simulink model "Diode_Clamped_Multilevel_Inverter"  (R2024a)
settings: Solver=FixedStepAuto  StartTime=0.0  StopTime=2/fe  FixedStep=1/(100*fsw)  RelTol=1e-3
values from neighbouring files (symbols this model uses):
  B = 0*0.0025    (= 0)    [ECE_598_script_file.m]
  fe = 100    [ECE_598_script_file.m]
  fsw = 1000    [ECE_598_script_file.m]
  J = 0.01    [ECE_598_script_file.m]
  Lrl_dash = 9.6e-3    (= 0.0096)    [ECE_598_script_file.m]
  Lsl = 9.6e-3    (= 0.0096)    [ECE_598_script_file.m]
  M = 165e-3    (= 0.165)    [ECE_598_script_file.m]
  Rr = 4.23    [ECE_598_script_file.m]
  Rs = 3.57    [ECE_598_script_file.m]
  tau_L = 2    [ECE_598_script_file.m]
  turns_ratio = 0.682    [ECE_598_script_file.m]
  Vdc = 400    [ECE_598_script_file.m]
  Vm = 200    [ECE_598_script_file.m]
undefined symbols (not defined in the file or in its folder): j, jsin
libraries: nesl_utility x23, ee_lib x20, fl_lib x12
(part 1 of 2)
settings Model: Creator=dm69  LastModifiedBy=dm69

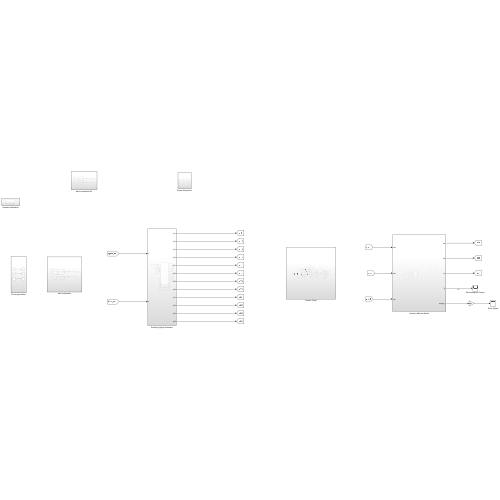
[thumbnail: Simulink's stored preview of the top-level diagram]
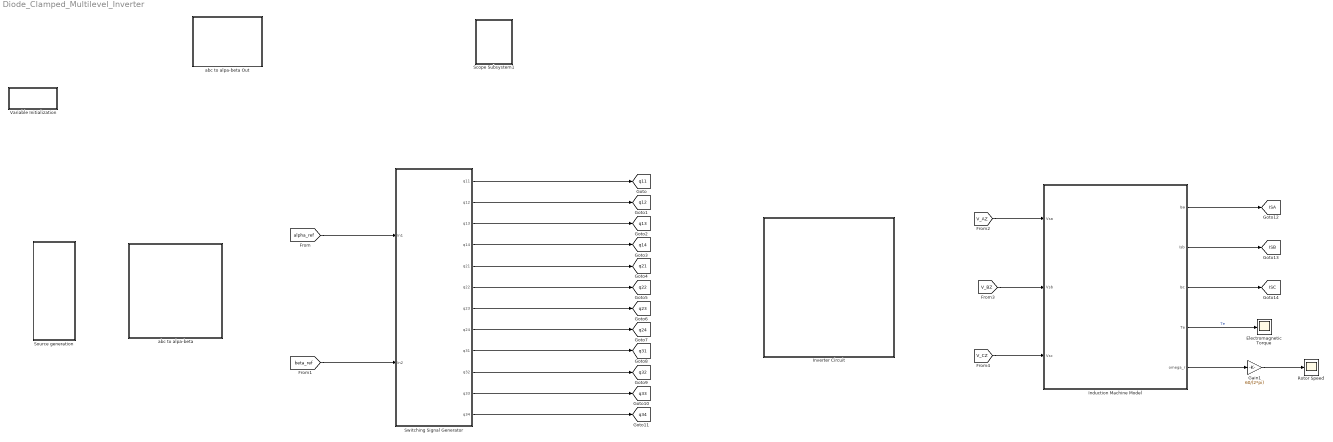
== system Diode_Clamped_Multilevel_Inverter ==
  Electromagnetic Torque : Scope
  Gain1 : Gain  Gain=60/(2*pi)
  Induction Machine Model : Subsystem
  Inverter Circuit : Subsystem
  Rotor Speed : Scope
  Scope Subsystem1 : Subsystem
  Source generation : Subsystem
  Switching Signal Generator : Subsystem
  Variable Initialization : Subsystem
  abc to alpa-beta : Subsystem
  abc to alpa-beta Out : Subsystem
  tag scope: ISA=global, ISB=global, ISC=global, q11=global, q12=global, q13=global, q14=global, q21=global, q22=global, q23=global, q24=global, q31=global, q32=global, q33=global, q34=global
  wires:
  Gain1/1 -> Rotor Speed/1
  Induction Machine Model/2(Isb) -> [ISB]
  Induction Machine Model/3(Isc) -> [ISC]
  Induction Machine Model/1(Isa) -> [ISA]
  Switching Signal Generator/11(q33) -> [q33]
  Switching Signal Generator/12(q34) -> [q34]
  Switching Signal Generator/10(q32) -> [q32]
  Switching Signal Generator/8(q24) -> [q24]
  Switching Signal Generator/9(q31) -> [q31]
  Switching Signal Generator/6(q22) -> [q22]
  Induction Machine Model/5(omega_r) -> Gain1/1
  Switching Signal Generator/3(q13) -> [q13]
  Switching Signal Generator/2(q12) -> [q12]
  Switching Signal Generator/1(q11) -> [q11]
  Switching Signal Generator/4(q14) -> [q14]
  Switching Signal Generator/5(q21) -> [q21]
  [alpha_ref] -> Switching Signal Generator/1(In1)
  Induction Machine Model/4(Te) -> Electromagnetic Torque/1  "Te"
  [beta_ref] -> Switching Signal Generator/2(In2)
  Switching Signal Generator/7(q23) -> [q23]
  [V_AZ] -> Induction Machine Model/1(Vsa)
  [V_BZ] -> Induction Machine Model/2(Vsb)
  [V_CZ] -> Induction Machine Model/3(Vsc)

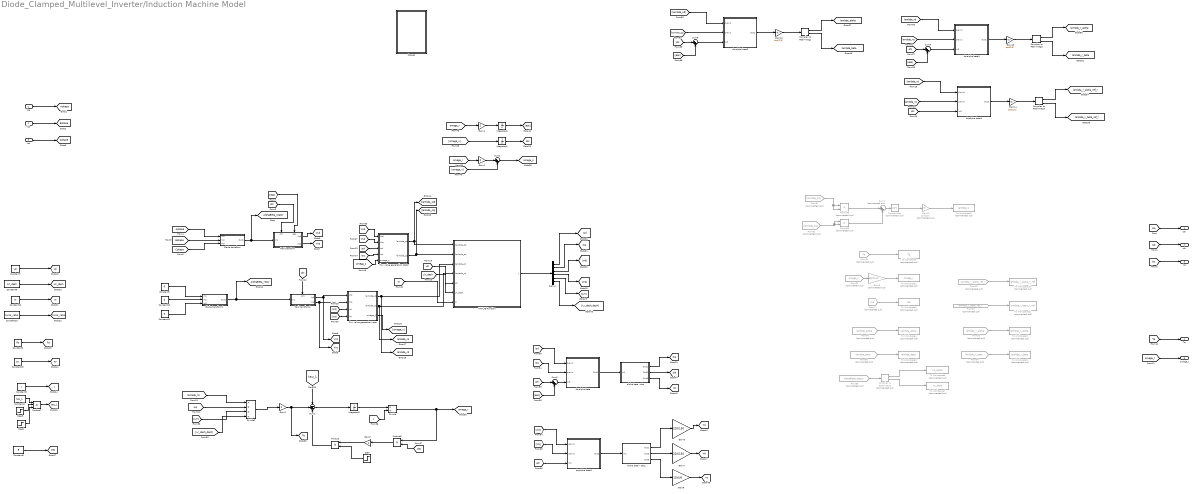
== system Diode_Clamped_Multilevel_Inverter/Induction Machine Model ==
  Vsa : Inport
  Vsb : Inport  Port=2
  Vsc : Inport  Port=3
  Clarke transform : Subsystem
  Clarke transform1 : Subsystem
  Complex to Real-Imag1 : ComplexToRealImag
  Complex to Real-Imag2 : ComplexToRealImag  Commented=on
  Complex to Real-Imag3 : ComplexToRealImag
  Complex to Real-Imag4 : ComplexToRealImag
  Constant10 : Constant  Value=0
  Constant11 : Constant  Value=0
  Constant12 : Constant  Value=M
  Constant13 : Constant  Value=turns_ratio
  Constant15 : Constant  Value=Rr
  Constant3 : Constant  Value=J
  Constant4 : Constant  Value=tau_L
  Constant5 : Constant  Value=Rs
  Constant6 : Constant  Value=B
  Constant7 : Constant  Value=Lsl
  Constant8 : Constant  Value=Lrl_dash
  Constant9 : Constant  Value=0
  Demux : Demux  Outputs=6
  Divide : Product  Inputs=*/
  Divide2 : Product  Inputs=***/
  From43 : From  Commented=on  GotoTag=lambda_r_alpha_ref_r  TagVisibility=global
  From61 : From  Commented=on  GotoTag=Te  TagVisibility=global
  From62 : From  Commented=on  GotoTag=omega_r
  From74 : From  Commented=on  GotoTag=Isa  TagVisibility=global
  From81 : From  Commented=on  GotoTag=lambda_sd
  From82 : From  Commented=on  GotoTag=lambda_sq
  From87 : From  Commented=on  GotoTag=lambda_alpha  TagVisibility=global
  From88 : From  Commented=on  GotoTag=lambda_beta  TagVisibility=global
  From89 : From  Commented=on  GotoTag=AlphaBeta_stator
  From92 : From  Commented=on  GotoTag=lambda_r_beta_ref_r  TagVisibility=global
  From93 : From  Commented=on  GotoTag=lambda_r_alpha  TagVisibility=global
  From94 : From  Commented=on  GotoTag=lambda_r_beta  TagVisibility=global
  Gain1 : Gain  Gain=2
  Gain11 : Gain  Commented=on  Gain=sqrt(2/3)
  Gain12 : Gain  Gain=sqrt(2/3)
  Gain13 : Gain  Gain=sqrt(2/3)
  Gain14 : Gain  Gain=sqrt(2/3)
  Gain2 : Gain  Gain=2
  Gain3 : Gain
  Gain4 : Gain  Gain=2
  Gain6 : Gain  Gain=220/150
  Gain7 : Gain  Gain=220/150
  Gain8 : Gain  Gain=220/150
  Gain9 : Gain  Commented=on  Gain=60/(2*pi)
  Integrator1 : Integrator  InitialCondition=1e-4
  Integrator3 : Integrator
  Integrator6 : Integrator  InitialCondition=1e-4
  MATLAB Function : MATLAB Function  TreatAsAtomicUnit=on
  Park transform : Subsystem
      settings: PortSchema="{\"entries\":[{\"content\":{\"sides\":[{\"content\":{\"connectorIds\":[\"In1\"]},\"type\":\"ConnectorPlacement.EquallySpacedRectSide\",\"uuid\":\"6c71d13c-178f-4a42-b33e-304e9d2b6e08\"},{\"content\":{\"connectorIds\":[\"Out1\",\"Out2\"],\"side\":\"RIGHT\"},\"type\":\"ConnectorPlacement.EquallySpacedRectSide\",\"uuid\":\"2a6462c8-5182-4726-b418-a85255dbc142\"},{\"content\":{\"connectorIds\":[\"In2\",\"In3\"],\"side\":\"TOP\"},\"type\":\"ConnectorPlacement.EquallySpacedRectSide\",\"uuid\":\"09083f92-b28e-408e-9b2d-669b336a5b1a\"}]},\"type\":\"ConnectorPlacement.EquallySpacedConnector\",\"uuid\":\"431009d8-f15a-4fdd-ac9b-0312528d9d69\"}],\"packageUris\":[\"http://schema.mathworks.com/mf0/Connector/R2020b\"],\"version\":\"1.0\"}"
  Park transform1 : Subsystem
      settings: PortSchema="{\"entries\":[{\"content\":{\"sides\":[{\"content\":{\"connectorIds\":[\"In1\"]},\"type\":\"ConnectorPlacement.EquallySpacedRectSide\",\"uuid\":\"6c71d13c-178f-4a42-b33e-304e9d2b6e08\"},{\"content\":{\"connectorIds\":[\"Out1\",\"Out2\"],\"side\":\"RIGHT\"},\"type\":\"ConnectorPlacement.EquallySpacedRectSide\",\"uuid\":\"2a6462c8-5182-4726-b418-a85255dbc142\"},{\"content\":{\"connectorIds\":[\"In2\"],\"side\":\"TOP\"},\"type\":\"ConnectorPlacement.EquallySpacedRectSide\",\"uuid\":\"09083f92-b28e-408e-9b2d-669b336a5b1a\"}]},\"type\":\"ConnectorPlacement.EquallySpacedConnector\",\"uuid\":\"431009d8-f15a-4fdd-ac9b-0312528d9d69\"}],\"packageUris\":[\"http://schema.mathworks.com/mf0/Connector/R2020b\"],\"version\":\"1.0\"}"
  Product : Product
  Product2 : Product
  Product7 : Product  Inputs=3
  Product8 : Product  Commented=on
  Product9 : Product  Commented=on
  Scopes : Subsystem
  Square Root : Sqrt  Commented=on
  Step : Step  Time=1e-3  SampleTime=0
  Step1 : Step  Time=8  Before=1  After=0  SampleTime=0
  Step3 : Step  Time=4  SampleTime=0
  Sum1 : Sum  Inputs=-+-
  Sum{2,5,8..9} (4 alike) : Sum  Inputs=|++
  Sum7 : Sum  Commented=on  Inputs=|++
  To Workspace : ToWorkspace  Commented=on  VariableName=Te  SaveFormat=Timeseries  SampleTime=-1
  To Workspace1 : ToWorkspace  Commented=on  VariableName=omega_r  SaveFormat=Timeseries  SampleTime=-1
  To Workspace10 : ToWorkspace  Commented=on  VariableName=lambda_r_alpha_r_ref  SaveFormat=Timeseries  SampleTime=-1
  To Workspace11 : ToWorkspace  Commented=on  VariableName=lambda_r_beta_r_ref  SaveFormat=Timeseries  SampleTime=-1
  To Workspace2 : ToWorkspace  Commented=on  VariableName=Isa  SaveFormat=Timeseries  SampleTime=-1
  To Workspace3 : ToWorkspace  Commented=on  VariableName=lambda_s  SaveFormat=Timeseries  SampleTime=-1
  To Workspace4 : ToWorkspace  Commented=on  VariableName=lambda_alpha  SaveFormat=Timeseries  SampleTime=-1
  To Workspace5 : ToWorkspace  Commented=on  VariableName=lambda_beta  SaveFormat=Timeseries  SampleTime=-1
  To Workspace6 : ToWorkspace  Commented=on  VariableName=Vs_alpha  SaveFormat=Timeseries  SampleTime=-1
  To Workspace7 : ToWorkspace  Commented=on  VariableName=Vs_beta  SaveFormat=Timeseries  SampleTime=-1
  To Workspace8 : ToWorkspace  Commented=on  VariableName=lambda_r_alpha  SaveFormat=Timeseries  SampleTime=-1
  To Workspace9 : ToWorkspace  Commented=on  VariableName=lambda_r_beta  SaveFormat=Timeseries  SampleTime=-1
  alpha beta - abc : Subsystem
  alpha beta - abc1 : Subsystem
  dq-alpha beta : Subsystem
  dq-alpha beta1 : Subsystem
  dq-alpha beta2 : Subsystem
  dq-alpha beta3 : Subsystem
  dq-alpha beta4 : Subsystem
  flux value generation rotor : Subsystem
  flux value generation stator : Subsystem
  Isa : Outport
  Isb : Outport  Port=2
  Isc : Outport  Port=3
  Te : Outport  Port=4
  omega_r : Outport  Port=5
  tag scope: AlphaBeta_rotor=global, AlphaBeta_stator=global, Aphase=global, Bphase=global, Cphase=global, Ira=global, Irb=global, Irc=global, Isa=global, Isb=global, Isc=global, Isd=global, Isq=global, J=global, Llr_dash=global, Lsl=global, M=global, Rr=global, Rs=global, Te=global, Vrd=global, Vrq=global, Vsd=global, Vsq=global, lambda_alpha=global, lambda_beta=global, lambda_r_alpha=global, lambda_r_alpha_ref_r=global, lambda_r_beta=global, lambda_r_beta_ref_r=global, lambda_rd=global, lambda_rq=global, omega_r=global, omega_s=global, phi=global, tau_L=global, turns_ratio=global
  wires:
  Gain4/1 -> Integrator6/1
  Clarke transform/1(Out1) -> [AlphaBeta_stator], Park transform/1(In1)
  Constant9/1 -> Clarke transform1/1(In1)
  From94/1 -> To Workspace9/1
  Demux/3 -> [Ird]
  Constant8/1 -> [Llr_dash]
  Constant11/1 -> Clarke transform1/3(In3)
  Integrator1/1 -> [phi]
  Clarke transform1/1(Out1) -> [AlphaBeta_rotor], Park transform1/1(In1)
  From61/1 -> To Workspace/1
  [phi] -> Sum9/1
  Demux/5 -> [Lm]
  Gain13/1 -> Complex to Real-Imag3/1
  Gain1/1 -> Sum2/1
  [Bphase] -> Clarke transform/2(In2)
  Gain9/1 -> To Workspace1/1
  flux value generation rotor/3(omega_X) -> [omega_x]
  [Isq] -> Divide2/2
  [M] -> MATLAB Function/7(M)
  Constant10/1 -> Clarke transform1/2(In2)
  flux value generation rotor/2(lambda_rq) -> MATLAB Function/4(lambda_rq), [lambda_rq]
  [lambda_rd] -> dq-alpha beta3/1(d-axis)
  dq-alpha beta/1(Out1) -> alpha beta - abc/1(In1)
  [Lr_dash_dash] -> Divide2/4
  [phi] -> dq-alpha beta1/3(In1)
  Constant15/1 -> [Rr]
  [Aphase] -> Clarke transform/1(In1)
  Complex to Real-Imag3/2 -> [lambda_r_beta]
  Integrator6/1 -> [eps]
  [Cphase] -> Clarke transform/3(In3)
  [Llr_dash] -> MATLAB Function/6(Lrl_dash)
  Sum9/1 -> dq-alpha beta3/3(In3)
  [omega_r] -> Gain1/1
  Gain6/1 -> [Ira]
  Park transform1/2(Vrq) -> [Vrq], flux value generation rotor/2(Vrq)
  Gain2/1 -> [Te], Sum1/2
  dq-alpha beta1/1(Out1) -> alpha beta - abc1/1(In1)
  alpha beta - abc1/1(Out1) -> Gain6/1
  [omega_s] -> flux value generation stator/5(omega_s)
  Constant5/1 -> [Rs]
  [lambda_rq] -> dq-alpha beta3/2(q-axis)
  flux value generation rotor/1(lambda_rd) -> MATLAB Function/3(lambda_rd), [lambda_rd]
  [eps] -> Park transform/3(eps)
  From81/1 -> Product8/2, Product8/1
  [J] -> Divide/2
  Sum1/1 -> Integrator3/1
  From88/1 -> To Workspace5/1
  Product7/1 -> [tau_L]
  [Lsl] -> MATLAB Function/5(Lsl)
  Demux/1 -> [Isd]
  Complex to Real-Imag4/2 -> [lambda_r_beta_ref_r]
  MATLAB Function/1(y) -> Demux/1
  alpha beta - abc/2(Out2) -> [Isb]
  [lambda_rd] -> Divide2/1
  Gain11/1 -> To Workspace3/1
  [B] -> Product2/2
  From93/1 -> To Workspace8/1
  Demux/2 -> [Isq]
  [Isd] -> flux value generation stator/3(Isd)
  [omega_r] -> Gain4/1
  flux value generation stator/1(lambda_sd) -> [lambda_sd], MATLAB Function/1(lambda_sd)
  [lambda_sd] -> dq-alpha beta2/1(d-axis)
  [Lm] -> Divide2/3
  Park transform1/1(Vrd) -> flux value generation rotor/1(Vrd), [Vrd]
  Constant13/1 -> [turns_ratio]
  [Ird] -> flux value generation rotor/3(Ird)
  Product8/1 -> Sum7/1
  From87/1 -> To Workspace4/1
  Product2/1 -> Gain3/1
  [Vsq] -> flux value generation stator/2(Vsq)
  Divide2/1 -> Gain2/1
  [phi] -> Sum5/1
  Constant3/1 -> [J]
  [eps] -> Sum5/2
  Gain7/1 -> [Irb]
  Constant7/1 -> [Lsl]
  Product9/1 -> Sum7/2
  Sum2/1 -> [omega_s]
  [tau_L] -> Sum1/1
  flux value generation stator/2(lambda_sq) -> [lambda_sq], MATLAB Function/2(lambda_sq)
  [phi] -> Park transform1/2(phi)
  [Irq] -> dq-alpha beta1/2(q-axis)
  Gain8/1 -> [Irc]
  [omega_x] -> Integrator1/1
  [Ird] -> dq-alpha beta1/1(d-axis)
  Constant12/1 -> [M]
  alpha beta - abc/1(Out1) -> [Isa]
  Square Root/1 -> Gain11/1
  alpha beta - abc1/3(Out3) -> Gain8/1
  [eps] -> Sum9/2
  Sum5/1 -> dq-alpha beta/3(In3)
  Park transform/2(Vsq) -> [Vsq]
  From74/1 -> To Workspace2/1
  [phi] -> Sum8/1
  Sum8/1 -> dq-alpha beta2/3(In3)
  Park transform/1(Vsd) -> [Vsd]
  Sum7/1 -> Square Root/1
  [Vsd] -> flux value generation stator/1(Vsd)
  From62/1 -> Gain9/1
  From89/1 -> Complex to Real-Imag2/1
  [omega_x] -> Sum2/2
  [eps] -> Sum8/2
  dq-alpha beta2/1(Out1) -> Gain12/1
  Complex to Real-Imag1/2 -> [lambda_beta]
  [Isd] -> dq-alpha beta/1(d-axis)
  Complex to Real-Imag2/1 -> To Workspace6/1
  Step3/1 -> Product7/2
  alpha beta - abc/3(Out3) -> [Isc]
  From82/1 -> Product9/1, Product9/2
  Complex to Real-Imag1/1 -> [lambda_alpha]
  [phi] -> Park transform/2(phi)
  Demux/4 -> [Irq]
  dq-alpha beta3/1(Out1) -> Gain13/1
  Gain12/1 -> Complex to Real-Imag1/1
  dq-alpha beta4/1(Out1) -> Gain14/1
  Divide/1 -> [omega_r], Product2/1
  [Isq] -> flux value generation stator/4(Isq)
  alpha beta - abc1/2(Out2) -> Gain7/1
  Gain14/1 -> Complex to Real-Imag4/1
  [lambda_rq] -> dq-alpha beta4/2(q-axis)
  [lambda_rd] -> dq-alpha beta4/1(d-axis)
  Integrator3/1 -> Divide/1
  Complex to Real-Imag3/1 -> [lambda_r_alpha]
  Demux/6 -> [Lr_dash_dash]
  [Irq] -> flux value generation rotor/4(Irq)
  Constant6/1 -> [B]
  Constant4/1 -> Product7/1
  Complex to Real-Imag2/2 -> To Workspace7/1
  [Isq] -> dq-alpha beta/2(q-axis)
  [lambda_sq] -> dq-alpha beta2/2(q-axis)
  From92/1 -> To Workspace11/1
  [phi] -> dq-alpha beta4/3(In3)
  Complex to Real-Imag4/1 -> [lambda_r_alpha_ref_r]
  From43/1 -> To Workspace10/1
  [Isa] -> Isa/1
  [Isb] -> Isb/1
  [Isc] -> Isc/1
  [Te] -> Te/1
  [omega_r] -> omega_r/1
  Vsa/1 -> [Aphase]
  Vsb/1 -> [Bphase]
  Vsc/1 -> [Cphase]
  Gain3/1 -> Product/1
  Product/1 -> Sum1/3
  Step/1 -> Product/2
  Step1/1 -> Product7/3

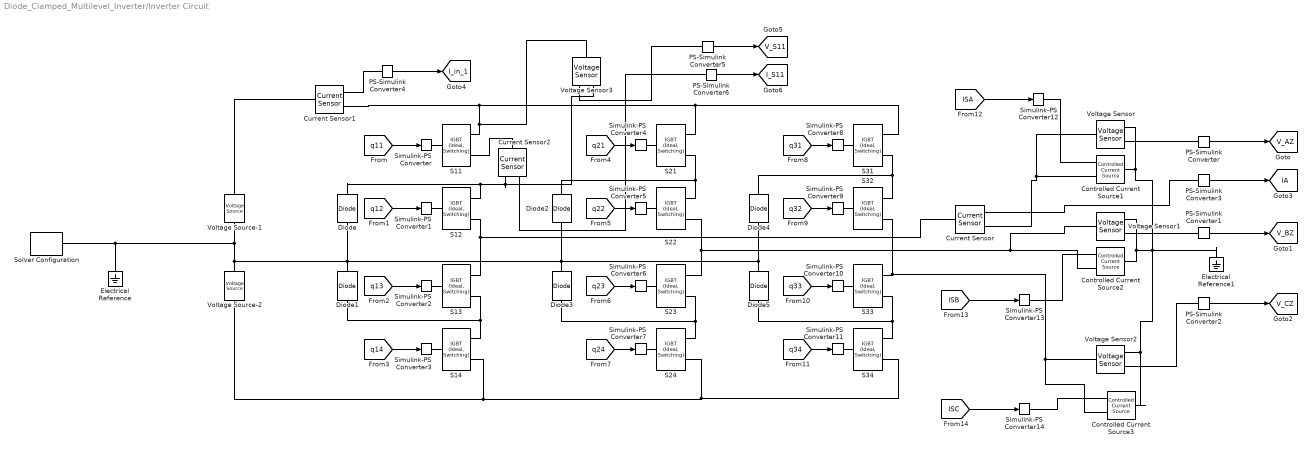
== system Diode_Clamped_Multilevel_Inverter/Inverter Circuit ==
  Controlled Current Source1 : fl_lib/Electrical/Electrical Sources/Controlled Current Source
  Controlled Current Source2 : fl_lib/Electrical/Electrical Sources/Controlled Current Source
  Controlled Current Source3 : fl_lib/Electrical/Electrical Sources/Controlled Current Source
  Current Sensor : fl_lib/Electrical/Electrical Sensors/Current Sensor
  Current Sensor1 : fl_lib/Electrical/Electrical Sensors/Current Sensor
  Current Sensor2 : fl_lib/Electrical/Electrical Sensors/Current Sensor
  Diode{,1..5} (6 alike) : ee_lib/Semiconductors & Converters/Diode  ModelType=ee.enum.diode.modelType.pwl  TableType=ee.enum.diode.tableType.IfMat  IfMat=[.07, .12, .19, 1.75, 4.24, 7.32, 11.2; .16, .3, .72, 2.14, 5.02, 8.35, 13.12] A  VfMat=[.9, 1.15, 1.25, 1.5, 1.75, 2.17, 2.6, 2.85; .58, .68, .75, 1.1, 1.38, 1.77, 2.27, 2.7] V  TjVec=[25, 125] degC  VfVec=[.5, .7, .9, 1.3, 1.7, 2.1, 2.5] V  IfVec=[.1, .2, .5, 1, 2, 4, 7, 10] A  IrMat=[1e-06, 2e-06, 5e-06, 1e-05, 2.5e-05, 5e-05, .0001; 2e-06, 5e-06, 1e-05, 4e-05, 8e-05, .0002, .0005] A  VrMat=[10, 100, 200, 250, 300, 325, 350; 10, 70, 160, 220, 270, 300, 320] V  VrVec=[10, 20, 40, 50, 70, 80, 100] V  IrVec=[1e-06, 2e-06, 5e-06, 1e-05, 2e-05, 5e-05, .0001] A  Vf=0.6 V  Ron=0.3 Ohm  Goff=1e-8 S  prmExp=ee.enum.diode.expParam.useTwo  I12=[.0137, .545] A  V12=[.6, .7] V  RS=0 Ohm  Tmeas=298.15 K  IS=1e-12 A  ec=1  I1=0.0137 A  V1=0.6 V  N_series=1  N_parallel=1  ZenerEnable=false  Rz=0.3 Ohm  BV=inf V  C_param=ee.enum.diode.capParam.fixed  CJ=0 pF  CJ0=5 pF  Vvec=[.1, 10, 100] V  Cvec=[3.5, 1, .4] pF  VJ=1 V  Mgrad=0.5  FC=0.5  Q_param=ee.enum.diode.recoveryParam.off  iRM=-7.15 A  iF=4 A  didt=-750 A/us  trr_factor=3  trr=115 ns  Qrr=150 nA*s  Vr=-600 V  Ls=150 nH  Erec=0.03 J  TT=50 ns  tau=100 ns  T_param=ee.enum.diode.temperatureParam.off  Tdevice=298.15 K  I1_T2=0.245 A  V1_T2=0.5 V  IS_T2=1.25e-7 A  Tmeas2=125 degC  XTI_param=ee.enum.diode.xtiParam.pn  XTI=3  EG_param=ee.enum.diode.egapParam.material_si  EG=1.11 eV  dBVdT=0 V/K  enable_faults=simscape.enum.onoff.off  fault_action=simscape.enum.assert.action.none  fault_types=ee.enum.diode.faults.open  tau_fault=1e-3 s  IfMat_faulted=[.07, .12, .19, 1.75, 4.24, 7.32, 11.2; .16, .3, .72, 2.14, 4.02, 6.35, 9.12] A  VfMat_faulted=[.9, 1.15, 1.25, 1.5, 1.75, 2.17, 2.6, 2.85; .58, .68, .75, 1.1, 1.38, 1.77, 2.27, 2.7] V  VfVec_faulted=[.5, .7, .9, 1.3, 1.7, 2.1, 2.5] V  IfVec_faulted=[.1, .2, .5, 1, 2, 4, 7, 10] A  IrMat_faulted=[1e-06, 2e-06, 5e-06, 1e-05, 2.5e-05, 5e-05, .0001; 2e-06, 5e-06, 1e-05, 4e-05, 8e-05, .0002, .0005] A  VrMat_faulted=[1, 10, 20, 25, 30, 32.5, 35; 1, 5, 10, 20, 25, 30, 32] V  VrVec_faulted=[1, 2, 4, 5, 7, 8, 10] V  IrVec_faulted=[1e-06, 2e-06, 5e-06, 1e-05, 2e-05, 5e-05, .0001] A  Ropen_faulted=1000 Ohm  Gshort_faulted=1000 1/Ohm  Vf_faulted=0.6 V  Ron_faulted=0.3 Ohm  Goff_faulted=1e-8 S  I12_faulted=[.0137, .545] A  V12_faulted=[.6, .7] V  IS_faulted=1e-12 A  ec_faulted=1  I1_faulted=0.0137 A  V1_faulted=0.6 V  RS_faulted=0 Ohm  Rz_faulted=0.3 Ohm  BV_faulted=inf V  Cscale_faulted=100  fault_trigger=ee.enum.faults.faultTrigger.temporal  t_fault=inf s  max_permissible_voltage=inf V  n_fail_on_voltage=1  max_permissible_current=inf A  t_fail_on_current=1 s  max_permissible_dVdt=inf V/s  enable_fault_input=simscape.enum.onoff.off  i_specify=off  i_priority=None  i=0 A  i_nominal_specify=off  i_nominal_value=1  i_nominal_unit=A  v_specify=off  v_priority=None  v=0 V  v_nominal_specify=off  v_nominal_value=1  v_nominal_unit=V  v_capacitor_specify=off  v_capacitor_priority=None  v_capacitor=0 V  v_capacitor_nominal_specify=off  v_capacitor_nominal_value=1  v_capacitor_nominal_unit=V  Qj_specify=off  Qj_priority=High  Qj=0 C  Qj_nominal_specify=off  Qj_nominal_value=1  Qj_nominal_unit=C  faulted_specify=off  faulted_priority=None  faulted=0  faulted_nominal_specify=off  faulted_nominal_value=1  faulted_nominal_unit=1  i_diode_specify=off  i_diode_priority=None  i_diode=0 A  i_diode_nominal_specify=off  i_diode_nominal_value=1  i_diode_nominal_unit=A  v_diode_specify=off  v_diode_priority=None  v_diode=0 V  v_diode_nominal_specify=off  v_diode_nominal_value=1  v_diode_nominal_unit=V  i_capacitor_specify=off  i_capacitor_priority=None  i_capacitor=0 A  i_capacitor_nominal_specify=off  i_capacitor_nominal_value=1  i_capacitor_nominal_unit=A  power_dissipated_specify=off  power_dissipated_priority=None  power_dissipated=0 W  power_dissipated_nominal_specify=off  power_dissipated_nominal_value=1  power_dissipated_nominal_unit=W  fidelity_level=ee.enum.diode.fidelity.includeChargeDyn  rec_loss_model=ee.enum.diode.reverseRecoveryModel.fixed  ErecVal=0 J  scaleWithIandV=true  ErecMat=zeros(2, 3) J  TjrecVec=[298.15, 398.15] K  IfrecVec=[.1, 1, 10] A  IrecVal=10 A  VrecVal=10 V  tFilter=1 / 1000 / 100 s  max_permissible_temperature=inf K  t_fail_on_temperature=1 s  thermal_network_parameterization=ee.enum.thermalNetworkTopology.junctionCase  Rth=[0, 10] K/W  Rth_Cauer=[1, 3, 10] K/W  Rth_Foster=[4, 6] K/W  thermal_mass_parameterization=ee.enum.thermalNetwork.timeconstant  thermal_mass=[0, 1] J/K  thermal_mass_Cauer=[.1, .3, 1] J/K  thermal_mass_Foster=[1.5, 3] J/K  thermal_time_constant=[0, 10] s  thermal_time_constant_Cauer=[1, 3, 10] s  thermal_time_constant_Foster=[6, 18] s  thermal_mass_initial_temperatures=[25, 25] degC  thermal_mass_initial_temperatures_Cauer=[25, 25, 25] degC  junction_thermal_mass=0.01 J/K  Tvec_initial_Foster=[25, 25, 25, 25] degC  no_thermal_network=0  junction_temperature_specify=off  junction_temperature_priority=None  junction_temperature=25 degC  junction_temperature_nominal_specify=off  junction_temperature_nominal_value=1  junction_temperature_nominal_unit=degC
  Electrical Reference : fl_lib/Electrical/Electrical Elements/Electrical Reference
  Electrical Reference1 : fl_lib/Electrical/Electrical Elements/Electrical Reference
  PS-Simulink Converter{,1..6} (7 alike) : nesl_utility/PS-Simulink Converter  PhysicalDomain=network_engine_domain  SubClassName=ps_output  LeftPortType=input  RightPortType=output  PseudoPeriodic=off  Frequencies=[]  VectorFormat=inherit  Unit=inherit  AffineConversion=off
  S{11..14,21..24,31..34} (12 alike) : ee_lib/Semiconductors & Converters/IGBT (Ideal, Switching)  port_option=ee.enum.controlport.ps  Vf=0.8 V  Ron=0.001 Ohm  Goff=1e-5 1/Ohm  Vth=6 V  diode_param=ee.enum.semiconductors.protectionDiode.nodynamics  diode_Vf=0.8 V  diode_Ron=0.001 Ohm  diode_Goff=1e-5 1/Ohm  diode_C=50e-9 F  diode_iRM=-235 A  diode_iF=300 A  diode_idot=-50 A/us  diode_trr_param=ee.enum.converters.diodeReverseParam.trr_factor  diode_trr_factor=3  diode_trr=15 us  diode_Qrr=1500 s*uA  ice_specify=off  ice_priority=None  ice=0 A  ice_nominal_specify=off  ice_nominal_value=1  ice_nominal_unit=A  vce_specify=off  vce_priority=None  vce=0 V  vce_nominal_specify=off  vce_nominal_value=1  vce_nominal_unit=V  vge_specify=off  vge_priority=None  vge=0 V  vge_nominal_specify=off  vge_nominal_value=1  vge_nominal_unit=V  thermal_loss_option=ee.enum.converters.thermalLossOption.constantvalues  Von_data=[0, .1, .6, .8, 1, 1.3, 1.6, 2, 2.4; 0, .1, .7, 1, 1.2, 1.5, 1.9, 2.4, 2.8] V  Tj=[298.15, 398.15] K  Iout_data=[0, .1, 1, 5, 10, 20, 40, 70, 100] A  Eon_data=[0, .0024, .024, .12, .2, .48, 1.04, 2.16, 3.24; 0, .003, .03, .15, .25, .6, 1.3, 2.7, 4.05] * 1e-3 J  Eoff_data=[0, .0007, .0066, .033, .066, .17, .33, .83, 1.5; 0, .001, .01, .05, .1, .25, .5, 1.2, 2.2] * 1e-3 J  Eon_data_3D=[zeros(2, 9, 3)] J  Eoff_data_3D=[zeros(2, 9, 3)] J  Tj_loss=[298.15, 398.15] K  Iout_data_loss=[0, .1, 1, 5, 10, 20, 40, 70, 100] A  tabulateWithVce=false  Vce_loss=[0, 150, 300] V  Eon_scalar=22.86e-3 J  Eoff_scalar=17.14e-3 J  Voff=300 V  Iout_scalar=600 A  useCurrentFromPreviousCycle=false  useVoltageFromPreviousCycle=false  diodeModelType=ee.enum.converters.diodeModelType.pwl  diodeTableType=ee.enum.diode.tableType.IfMat  diode_ReverseIVType=ee.enum.diode.diodeReverseIV.constant  diode_IfMat=[.07, .12, .19, 1.75, 4.24, 7.32, 11.2; .16, .3, .72, 2.14, 4.02, 6.35, 9.12] A  diode_VfMat=[.9, 1.15, 1.25, 1.5, 1.75, 2.17, 2.6, 2.85; .58, .68, .75, 1.1, 1.38, 1.77, 2.27, 2.7] V  diode_TjVec=[25, 125] degC  diode_VfVec=[.5, .7, .9, 1.3, 1.7, 2.1, 2.5] V  diode_IfVec=[.1, .2, .5, 1, 2, 4, 7, 10] A  diode_IrMat=[1e-06, 2e-06, 5e-06, 1e-05, 2.5e-05, 5e-05, .0001; 2e-06, 5e-06, 1e-05, 4e-05, 8e-05, .0002, .0005] A  diode_VrMat=[10, 100, 200, 250, 300, 325, 350; 10, 70, 160, 220, 270, 300, 320] V  diode_VrVec=[10, 20, 40, 50, 70, 80, 100] V  diode_IrVec=[1e-06, 2e-06, 5e-06, 1e-05, 2e-05, 5e-05, .0001] A  diode_Vr=-600 V  diode_Ls=150 nH  diode_Erec=0.03 J  diode_rec_loss_model=ee.enum.diode.reverseRecoveryModel.fixed  diode_ErecVal=0 J  diode_scaleWithIandV=true  diode_ErecMat=zeros(2, 3) J  diode_TjrecVec=[298.15, 398.15] K  diode_IfrecVec=[.1, 1, 10] A  diode_IrecVal=10 A  diode_VrecVal=10 V  diode_tFilter=1 / 1000 / 100 s  thermal_network_parameterization=ee.enum.thermalNetworkTopology.external  Rth=[.08, .5] K/W  Rth_Cauer=[.08, .1, .5] K/W  Rth_Foster=[.08, .14, .22, .16] K/W  thermal_mass_parameterization=ee.enum.thermalNetwork.timeconstant  thermal_mass=[.01, .5] J/K  thermal_mass_Cauer=[.01, .1, .5] J/K  thermal_mass_Foster=[.001, .005, .05, .5] J/K  thermal_time_constant=[.001, .2] s  thermal_time_constant_Cauer=[.001, .1, .2] s  thermal_time_constant_Foster=[7e-05, .0007, .01, .08] s  thermal_mass_initial_temperatures=[25, 25] degC  thermal_mass_initial_temperatures_Cauer=[25, 25, 25] degC  junction_thermal_mass=0.01 J/K  Tvec_initial_Foster=[25, 25, 25, 25] degC  no_thermal_network=0  junction_temperature_specify=off  junction_temperature_priority=None  junction_temperature=25 degC  junction_temperature_nominal_specify=off  junction_temperature_nominal_value=1  junction_temperature_nominal_unit=degC  Qj_specify=off  Qj_priority=None  Qj=0 W  Qj_nominal_specify=off  Qj_nominal_value=1  Qj_nominal_unit=W  accumulatedSwitchingLosses_specify=off  accumulatedSwitchingLosses_priority=None  accumulatedSwitchingLosses=0 J
  Simulink-PS Converter{,1..14} (15 alike) : nesl_utility/Simulink-PS Converter  PhysicalDomain=network_engine_domain  SubClassName=ps_input  LeftPortType=input  RightPortType=output  PseudoPeriodic=off  Frequencies=[]  NoiseDistribution=none  NoiseParameters=[]  Unit=1  AffineConversion=off  FilteringAndDerivatives=provide  SimscapeFilterOrder=1  InputFilterTimeConstant=0.001  UdotUserProvided=0
  Solver Configuration : nesl_utility/Solver Configuration  PhysicalDomain=network_engine_domain  SubClassName=solver  LeftPortType=input  RightPortType=generic  Tones=[]  Harmonics=[]  SimulateNoise=off  Profile=off  UseLocalSampling=off  EnableSwitchedLinearOptims=on  FrequencyDomain=off  UseCCode=off  RelTol=0.001  AbsTol=0.001  MinStep=1e-09  ToWorkspace=off  RevertToSquareIcSolve=off  NumHomotopyIterations=100  PhasorMode=off  PhasorModeNumHarmonics=1  ConsistencySolver=NEWTON_XTOL_AFTER_FTOL  IndexReductionMethod=DerivativeReplacement  DoDC=off  ResidualTolerance=1e-09  ConsistencyTolSource=GLOBAL  ConsistencyAbsTol=0.001  ConsistencyRelTol=0.001  ConsistencyTolFactor=0.001  UseLocalSolver=off  LocalSolverChoice=NE_BACKWARD_EULER_ADVANCER  ResolveIndetEquations=on  FunctionEvalNumThread=1  LocalSolverSampleTime=0.001  DoFixedCost=off  MaxNonlinIter=3  MaxModeIter=2  ComputeImpulses=off  ImpulseIterations=2  LinearAlgebra=auto  LinearAlgebraNumThread=0  EquationFormulation=NE_TIME_EF  DelaysMemoryBudget=1024  AutomaticFiltering=on  FilteringTimeConstant=0.001  PartitionStorageMethod=AS_NEEDED  PartitionMemoryBudget=1024  PartitionMethod=ROBUST  MultibodyUseLocalSolver=off  MultibodyLocalSolverChoice=ODE1  MultibodyLocalSolverSampleTime=0.001
  Voltage Sensor{,1..3} (4 alike) : fl_lib/Electrical/Electrical Sensors/Voltage Sensor
  Voltage Source-1 : ee_lib/Sources/Voltage Source  dc_voltage=Vdc/2 V  ac_voltage=0 V  ac_shift=0 rad  ac_frequency=60 Hz  noise_mode=ee.enum.sources.noise.Disabled  PSD=0 V^2/Hz  sample_time=1e-3 s  repeatability=ee.enum.sources.repeatability.NotRepeatable  user_seed=0  auto_seed=3922919431  i_specify=off  i_priority=None  i=0 A  i_nominal_specify=off  i_nominal_value=1  i_nominal_unit=A  v_specify=off  v_priority=None  v=0 V  v_nominal_specify=off  v_nominal_value=1  v_nominal_unit=V
  Voltage Source-2 : ee_lib/Sources/Voltage Source  dc_voltage=Vdc/2 V  ac_voltage=0 V  ac_shift=0 rad  ac_frequency=60 Hz  noise_mode=ee.enum.sources.noise.Disabled  PSD=0 V^2/Hz  sample_time=1e-3 s  repeatability=ee.enum.sources.repeatability.NotRepeatable  user_seed=0  auto_seed=2715962282  i_specify=off  i_priority=None  i=0 A  i_nominal_specify=off  i_nominal_value=1  i_nominal_unit=A  v_specify=off  v_priority=None  v=0 V  v_nominal_specify=off  v_nominal_value=1  v_nominal_unit=V
  tag scope: IA=global, I_S11=global, I_in_1=global, V_AZ=global, V_BZ=global, V_CZ=global, V_S11=global
  wires:
  [q11] -> Simulink-PS Converter/1
  [q12] -> Simulink-PS Converter1/1
  [q13] -> Simulink-PS Converter2/1
  [q14] -> Simulink-PS Converter3/1
  [q21] -> Simulink-PS Converter4/1
  [q34] -> Simulink-PS Converter11/1
  [q32] -> Simulink-PS Converter9/1
  [q31] -> Simulink-PS Converter8/1
  PS-Simulink Converter/1 -> [V_AZ]
  PS-Simulink Converter1/1 -> [V_BZ]
  PS-Simulink Converter2/1 -> [V_CZ]
  [q22] -> Simulink-PS Converter5/1
  [q23] -> Simulink-PS Converter6/1
  [q24] -> Simulink-PS Converter7/1
  [q33] -> Simulink-PS Converter10/1
  PS-Simulink Converter3/1 -> [IA]
  PS-Simulink Converter4/1 -> [I_in_1]
  [ISA] -> Simulink-PS Converter12/1
  [ISB] -> Simulink-PS Converter13/1
  [ISC] -> Simulink-PS Converter14/1
  PS-Simulink Converter5/1 -> [V_S11]
  PS-Simulink Converter6/1 -> [I_S11]
  connections:
  Diode/RConn1 -- Current Sensor2/RConn2 -- Voltage Sensor3/RConn2 -- S12/RConn1
  S13/RConn2 -- Diode1/LConn1 -- S14/RConn1
  Simulink-PS Converter/RConn1 -- S11/LConn1
  S12/LConn1 -- Simulink-PS Converter1/RConn1
  S14/LConn1 -- Simulink-PS Converter3/RConn1
  Simulink-PS Converter2/RConn1 -- S13/LConn1
  S14/RConn2 -- S34/RConn2 -- S24/RConn2 -- Voltage Source-2/RConn1
  S24/LConn1 -- Simulink-PS Converter7/RConn1
  S22/LConn1 -- Simulink-PS Converter5/RConn1
  Simulink-PS Converter4/RConn1 -- S21/LConn1
  Simulink-PS Converter6/RConn1 -- S23/LConn1
  S34/LConn1 -- Simulink-PS Converter11/RConn1
  S32/LConn1 -- Simulink-PS Converter9/RConn1
  Simulink-PS Converter8/RConn1 -- S31/LConn1
  Simulink-PS Converter10/RConn1 -- S33/LConn1
  S21/RConn2 -- Diode2/RConn1 -- S22/RConn1
  Voltage Sensor1/LConn1 -- S22/RConn2 -- S23/RConn1 -- Controlled Current Source2/RConn2
  S23/RConn2 -- Diode3/LConn1 -- S24/RConn1
  S12/RConn2 -- S13/RConn1 -- Current Sensor/LConn1
  S31/RConn2 -- Diode4/RConn1 -- S32/RConn1
  Voltage Sensor2/LConn1 -- S32/RConn2 -- S33/RConn1 -- Controlled Current Source3/RConn2
  S33/RConn2 -- Diode5/LConn1 -- S34/RConn1
  Voltage Sensor1/RConn2 -- Controlled Current Source2/LConn1 -- Controlled Current Source1/LConn1 -- Voltage Sensor/RConn2 -- Electrical Reference1/LConn1 -- Voltage Sensor2/RConn2 -- Controlled Current Source3/LConn1
  PS-Simulink Converter/LConn1 -- Voltage Sensor/RConn1
  PS-Simulink Converter1/LConn1 -- Voltage Sensor1/RConn1
  PS-Simulink Converter2/LConn1 -- Voltage Sensor2/RConn1
  S31/RConn1 -- Current Sensor1/RConn2 -- Voltage Sensor3/LConn1 -- S11/RConn1 -- S21/RConn1
  Solver Configuration/RConn1 -- Electrical Reference/LConn1 -- Diode4/LConn1 -- Diode5/RConn1 -- Diode2/LConn1 -- Diode3/RConn1 -- Diode/LConn1 -- Diode1/RConn1 -- Voltage Source-2/LConn1 -- Voltage Source-1/RConn1
  Current Sensor/RConn2 -- Voltage Sensor/LConn1 -- Controlled Current Source1/RConn2
  Current Sensor/RConn1 -- PS-Simulink Converter3/LConn1
  Voltage Source-1/LConn1 -- Current Sensor1/LConn1
  Current Sensor1/RConn1 -- PS-Simulink Converter4/LConn1
  Simulink-PS Converter12/RConn1 -- Controlled Current Source1/RConn1
  Simulink-PS Converter13/RConn1 -- Controlled Current Source2/RConn1
  Simulink-PS Converter14/RConn1 -- Controlled Current Source3/RConn1
  Voltage Sensor3/RConn1 -- PS-Simulink Converter5/LConn1
  S11/RConn2 -- Current Sensor2/LConn1
  Current Sensor2/RConn1 -- PS-Simulink Converter6/LConn1

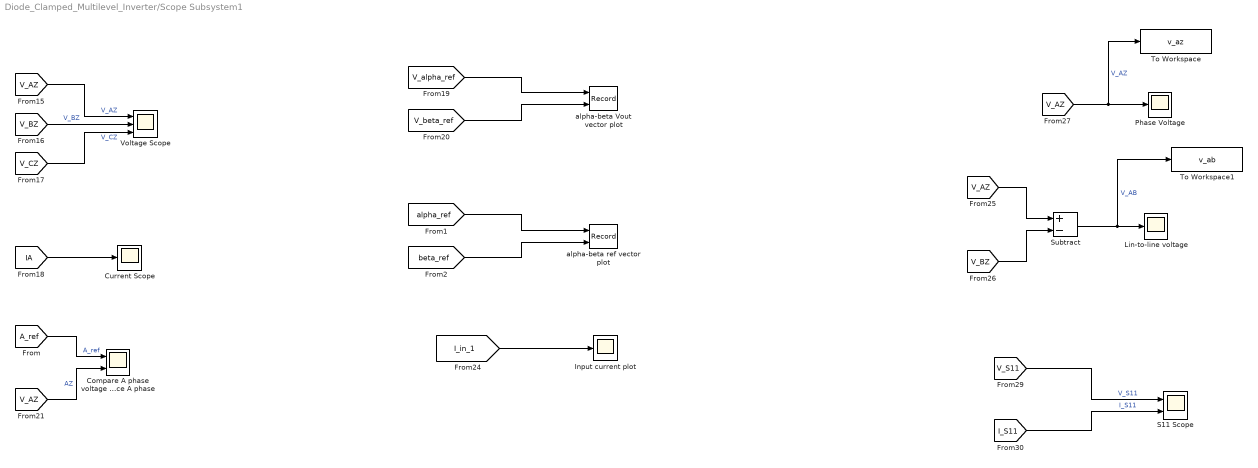
== system Diode_Clamped_Multilevel_Inverter/Scope Subsystem1 ==
  Compare A phase voltage with reference A phase : Scope  NumInputPorts=2
  Current Scope : Scope
  Input current plot : Scope
  Lin-to-line voltage : Scope
  Phase Voltage : Scope
  S11 Scope : Scope  NumInputPorts=2
  Subtract : Sum  Inputs=+-
  To Workspace : ToWorkspace  VariableName=v_az  SampleTime=-1
  To Workspace1 : ToWorkspace  VariableName=v_ab  SampleTime=-1
  Voltage Scope : Scope  NumInputPorts=3
  alpha-beta Vout vector plot : Record  FileSettingsInternal="{\"entries\":[{\"content\":{\"excelSettings\":{\"content\":{},\"type\":\"Streamout.ExcelSettings\"}},\"type\":\"Streamout.FileSettingStorage\",\"uuid\":\"\"}],\"packageUris\":[\"http:\\/\\/schema.mathworks.com\\/mf0\\/streamout_blocks\\/R2020a\"],\"version\":\"1.0\"}"  Layout=[1 1]  SignalsInternal="{\"entries\":[{\"content\":{\"signals\":[{\"content\":{\"blockPath\":[],\"dimensions\":[1],\"domain\":\"\",\"lineColor\":\"#a2142f\",\"plots\":[ 1 ],\"port\":1,\"signalID\":1,\"signalName\":\"From19\"},\"type\":\"RecordBlkView.Signal\",\"uuid\":\"\"},{\"content\":{\"blockPath\":[],\"dimensions\":[1],\"domain\":\"\",\"lineColor\":\"#139fff\",\"plots\":[ 1 ],\"port\":2,\"signalID\":2,\"signalName\":\"From20\"},\"type\":\"RecordBlkView.Signal\",\"uuid\":\"\"}]},\"type\":\"RecordBlkView.InputSignals\",\"uuid\":\"\"}],\"packageUris\":[\"http:\\/\\/schema.mathworks.com\\/mf0\\/streamout_blocks\\/R2020a\"],\"version\":\"1.0\"}"  VisualizationBindings="{\"xyplotplugin\":{\"info\":[{\"series\":[{\"bindingParametersList\":[{\"parameter\":\"X-Axis\",\"signalID\":1,\"signalName\":\"From19\"},{\"parameter\":\"Y-Axis\",\"signalID\":2,\"signalName\":\"From20\"}],\"seriesID\":0}],\"subplotID\":1}]}}"  CompatibilityTag=XY
  alpha-beta ref vector plot : Record  FileSettingsInternal="{\"entries\":[{\"content\":{\"excelSettings\":{\"content\":{},\"type\":\"Streamout.ExcelSettings\"}},\"type\":\"Streamout.FileSettingStorage\",\"uuid\":\"\"}],\"packageUris\":[\"http:\\/\\/schema.mathworks.com\\/mf0\\/streamout_blocks\\/R2020a\"],\"version\":\"1.0\"}"  Layout=[1 1]  SignalsInternal="{\"entries\":[{\"content\":{\"signals\":[{\"content\":{\"blockPath\":[],\"dimensions\":[1],\"domain\":\"\",\"lineColor\":\"#a2142f\",\"plots\":[ 1 ],\"port\":1,\"signalID\":1,\"signalName\":\"From1\"},\"type\":\"RecordBlkView.Signal\",\"uuid\":\"\"},{\"content\":{\"blockPath\":[],\"dimensions\":[1],\"domain\":\"\",\"lineColor\":\"#139fff\",\"plots\":[ 1 ],\"port\":2,\"signalID\":2,\"signalName\":\"From2\"},\"type\":\"RecordBlkView.Signal\",\"uuid\":\"\"}]},\"type\":\"RecordBlkView.InputSignals\",\"uuid\":\"\"}],\"packageUris\":[\"http:\\/\\/schema.mathworks.com\\/mf0\\/streamout_blocks\\/R2020a\"],\"version\":\"1.0\"}"  VisualizationBindings="{\"xyplotplugin\":{\"info\":[{\"series\":[{\"bindingParametersList\":[{\"parameter\":\"X-Axis\",\"signalID\":1,\"signalName\":\"From1\"},{\"parameter\":\"Y-Axis\",\"signalID\":2,\"signalName\":\"From2\"}],\"seriesID\":0}],\"subplotID\":1}]}}"  CompatibilityTag=XY
  wires:
  [alpha_ref] -> alpha-beta ref vector plot/1
  [beta_ref] -> alpha-beta ref vector plot/2
  [V_AZ] -> Voltage Scope/1  "V_AZ"
  [V_BZ] -> Voltage Scope/2  "V_BZ"
  [V_CZ] -> Voltage Scope/3  "V_CZ"
  [IA] -> Current Scope/1
  [V_beta_ref] -> alpha-beta Vout vector plot/2
  [V_alpha_ref] -> alpha-beta Vout vector plot/1
  [A_ref] -> Compare A phase voltage with reference A phase/1  "A_ref"
  [V_AZ] -> Compare A phase voltage with reference A phase/2  "AZ"
  [I_in_1] -> Input current plot/1
  [V_AZ] -> To Workspace/1, Phase Voltage/1  "V_AZ"
  [V_BZ] -> Subtract/2
  [V_AZ] -> Subtract/1
  Subtract/1 -> To Workspace1/1, Lin-to-line voltage/1  "V_AB"
  [V_S11] -> S11 Scope/1  "V_S11"
  [I_S11] -> S11 Scope/2  "I_S11"

== system Diode_Clamped_Multilevel_Inverter/Source generation ==
  A-phase : Sin  Amplitude=Vm  Frequency=2*pi*fe  SampleTime=0
  B-phase : Sin  Amplitude=Vm  Frequency=2*pi*fe  Phase=-2*pi/3  SampleTime=0
  C-phase : Sin  Amplitude=Vm  Frequency=2*pi*fe  Phase=-4*pi/3  SampleTime=0
  tag scope: A_ref=global, B_ref=global, C_ref=global
  wires:
  B-phase/1 -> [B_ref]
  C-phase/1 -> [C_ref]
  A-phase/1 -> [A_ref]

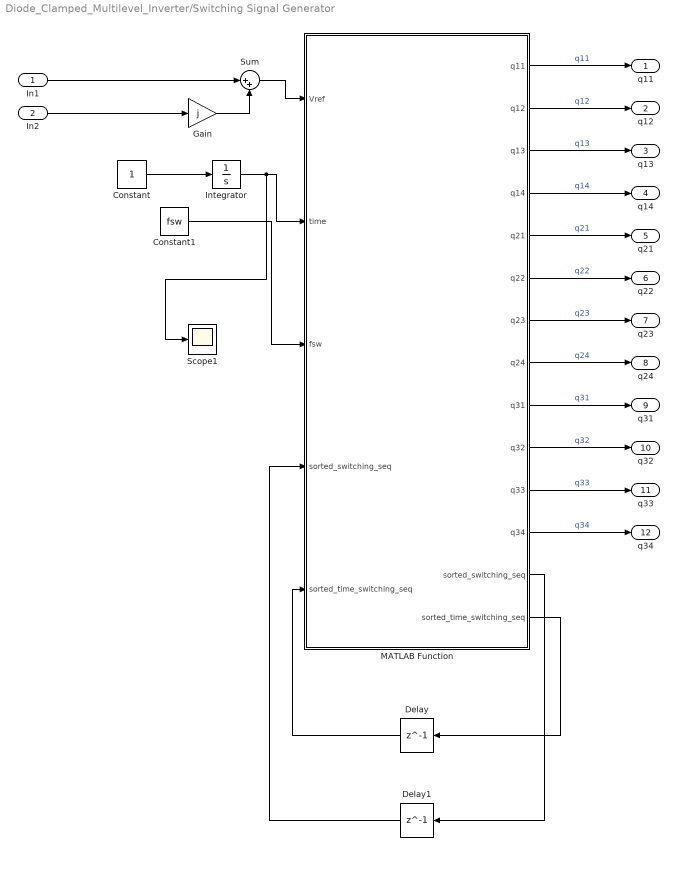
== system Diode_Clamped_Multilevel_Inverter/Switching Signal Generator ==
  In1 : Inport
  In2 : Inport  Port=2
  Constant : Constant
  Constant1 : Constant  Value=fsw
  Delay : Delay  DelayLength=1  InitialCondition=[0 0 0 0 0 0]  SampleTime=1/(100*fsw)
  Delay1 : Delay  DelayLength=1  InitialCondition=[0 0 0; 0 0 0; 0 0 0; 0 0 0; 0 0 0; 0 0 0]  SampleTime=1/(100*fsw)
  Gain : Gain  Gain=j
  Integrator : Integrator
  MATLAB Function : MATLAB Function  TreatAsAtomicUnit=on
  Scope1 : Scope
  Sum : Sum  Inputs=|++
  q11 : Outport
  q12 : Outport  Port=2
  q13 : Outport  Port=3
  q14 : Outport  Port=4
  q21 : Outport  Port=5
  q22 : Outport  Port=6
  q23 : Outport  Port=7
  q24 : Outport  Port=8
  q31 : Outport  Port=9
  q32 : Outport  Port=10
  q33 : Outport  Port=11
  q34 : Outport  Port=12
  wires:
  Constant/1 -> Integrator/1
  MATLAB Function/14(sorted_time_switching_seq) -> Delay/1
  Gain/1 -> Sum/2
  Constant1/1 -> MATLAB Function/3(fsw)
  Delay1/1 -> MATLAB Function/4("sorted_switching_seq ")
  Integrator/1 -> Scope1/1, MATLAB Function/2(time)
  MATLAB Function/13(sorted_switching_seq) -> Delay1/1
  MATLAB Function/6(q22) -> q22/1  "q22"
  Sum/1 -> MATLAB Function/1(Vref)
  Delay/1 -> MATLAB Function/5("sorted_time_switching_seq ")
  MATLAB Function/4(q14) -> q14/1  "q14"
  In1/1 -> Sum/1
  MATLAB Function/5(q21) -> q21/1  "q21"
  MATLAB Function/1(q11) -> q11/1  "q11"
  MATLAB Function/10(q32) -> q32/1  "q32"
  MATLAB Function/2(q12) -> q12/1  "q12"
  MATLAB Function/8(q24) -> q24/1  "q24"
  MATLAB Function/3(q13) -> q13/1  "q13"
  MATLAB Function/9(q31) -> q31/1  "q31"
  MATLAB Function/11(q33) -> q33/1  "q33"
  In2/1 -> Gain/1
  MATLAB Function/7(q23) -> q23/1  "q23"
  MATLAB Function/12(q34) -> q34/1  "q34"

== system Diode_Clamped_Multilevel_Inverter/Variable Initialization ==
  Constant : Constant  Value=fsw
  Constant1 : Constant  Value=Vm
  tag scope: Vm=global, fsw=global
  wires:
  Constant/1 -> [fsw]
  Constant1/1 -> [Vm]

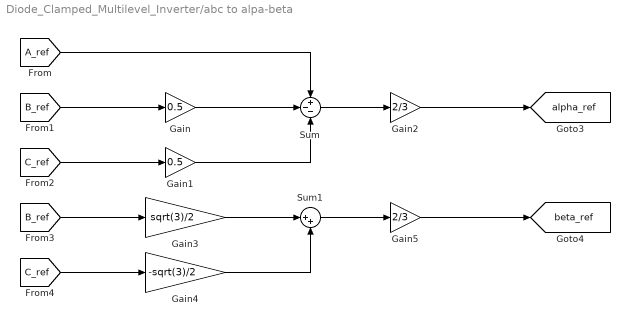
== system Diode_Clamped_Multilevel_Inverter/abc to alpa-beta ==
  Gain : Gain  Gain=0.5
  Gain1 : Gain  Gain=0.5
  Gain2 : Gain  Gain=2/3
  Gain3 : Gain  Gain=sqrt(3)/2
  Gain4 : Gain  Gain=-sqrt(3)/2
  Gain5 : Gain  Gain=2/3
  Sum : Sum  Inputs=+--
  Sum1 : Sum  Inputs=|++
  tag scope: alpha_ref=global, beta_ref=global
  wires:
  [A_ref] -> Sum/1
  [B_ref] -> Gain/1
  Gain/1 -> Sum/2
  [C_ref] -> Gain1/1
  Gain1/1 -> Sum/3
  Sum/1 -> Gain2/1
  Gain2/1 -> [alpha_ref]
  Gain3/1 -> Sum1/1
  [B_ref] -> Gain3/1
  [C_ref] -> Gain4/1
  Gain4/1 -> Sum1/2
  Sum1/1 -> Gain5/1
  Gain5/1 -> [beta_ref]

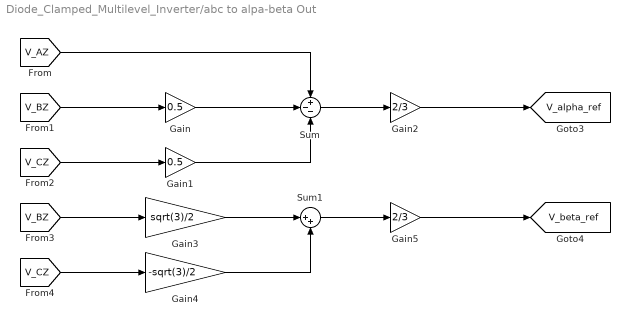
== system Diode_Clamped_Multilevel_Inverter/abc to alpa-beta Out ==
  Gain : Gain  Gain=0.5
  Gain1 : Gain  Gain=0.5
  Gain2 : Gain  Gain=2/3
  Gain3 : Gain  Gain=sqrt(3)/2
  Gain4 : Gain  Gain=-sqrt(3)/2
  Gain5 : Gain  Gain=2/3
  Sum : Sum  Inputs=+--
  Sum1 : Sum  Inputs=|++
  tag scope: V_alpha_ref=global, V_beta_ref=global
  wires:
  [V_AZ] -> Sum/1
  [V_BZ] -> Gain/1
  Gain/1 -> Sum/2
  [V_CZ] -> Gain1/1
  Gain1/1 -> Sum/3
  Sum/1 -> Gain2/1
  Gain2/1 -> [V_alpha_ref]
  Gain3/1 -> Sum1/1
  [V_BZ] -> Gain3/1
  [V_CZ] -> Gain4/1
  Gain4/1 -> Sum1/2
  Sum1/1 -> Gain5/1
  Gain5/1 -> [V_beta_ref]

== system Diode_Clamped_Multilevel_Inverter/Induction Machine Model/Clarke transform ==
  In1 : Inport
  In2 : Inport  Port=2
  In3 : Inport  Port=3
  Gain : Gain
  Gain1 : Gain  Gain=-0.5
  Gain2 : Gain  Gain=-0.5
  Gain3 : Gain  Gain=0
  Gain4 : Gain  Gain=0.866
  Gain5 : Gain  Gain=-0.866
  Gain6 : Gain  Gain=1j
  Gain7 : Gain  Gain=0.8165
  Sum : Sum  Inputs=+++
  Sum1 : Sum  Inputs=+++
  Sum2 : Sum  Inputs=|++
  Out1 : Outport
  wires:
  In1/1 -> Gain3/1, Gain/1  "A"
  Gain/1 -> Sum/1
  In2/1 -> Gain1/1, Gain4/1  "B"
  In3/1 -> Gain2/1, Gain5/1  "C"
  Gain1/1 -> Sum/2
  Gain3/1 -> Sum1/1
  Gain4/1 -> Sum1/2
  Gain5/1 -> Sum1/3
  Sum2/1 -> Gain7/1  "Vs_vec"
  Sum/1 -> Sum2/1  "alpha"
  Sum1/1 -> Gain6/1  "beta"
  Gain6/1 -> Sum2/2
  Gain7/1 -> Out1/1
  Gain2/1 -> Sum/3

== system Diode_Clamped_Multilevel_Inverter/Induction Machine Model/Clarke transform1 ==
  In1 : Inport
  In2 : Inport  Port=2
  In3 : Inport  Port=3
  Gain : Gain
  Gain1 : Gain  Gain=-0.5
  Gain2 : Gain  Gain=-0.5
  Gain3 : Gain  Gain=0
  Gain4 : Gain  Gain=0.866
  Gain5 : Gain  Gain=-0.866
  Gain6 : Gain  Gain=1j
  Gain7 : Gain  Gain=0.8165
  Sum : Sum  Inputs=+++
  Sum1 : Sum  Inputs=+++
  Sum2 : Sum  Inputs=|++
  Out1 : Outport
  wires:
  In1/1 -> Gain3/1, Gain/1  "A"
  Gain/1 -> Sum/1
  In2/1 -> Gain4/1, Gain1/1  "B"
  In3/1 -> Gain5/1, Gain2/1  "C"
  Gain1/1 -> Sum/2
  Gain2/1 -> Sum/3
  Gain3/1 -> Sum1/1
  Gain4/1 -> Sum1/2
  Gain5/1 -> Sum1/3
  Sum2/1 -> Gain7/1  "Vs_vec"
  Sum/1 -> Sum2/1  "alpha"
  Sum1/1 -> Gain6/1  "beta"
  Gain6/1 -> Sum2/2
  Gain7/1 -> Out1/1

== system Diode_Clamped_Multilevel_Inverter/Induction Machine Model/Park transform ==
  In1 : Inport
  phi : Inport  Port=2
  eps : Inport  Port=3
  Complex to Real-Imag : ComplexToRealImag
  Constant : Constant  Value=-pi/2
  Cos+jSin : Trigonometry  Operator=cos + jsin
  Gain : Gain  Gain=-1
  Product : Product
  Sum : Sum  Inputs=+++
  Vsd : Outport
  Vsq : Outport  Port=2
  wires:
  eps/1 -> Sum/2
  Sum/1 -> Gain/1
  In1/1 -> Product/1  "alpha-beta"
  Cos+jSin/1 -> Product/2
  Gain/1 -> Cos+jSin/1
  Complex to Real-Imag/1 -> Vsd/1  "d-axis"
  Complex to Real-Imag/2 -> Vsq/1  "q-axis"
  phi/1 -> Sum/1
  Constant/1 -> Sum/3
  Product/1 -> Complex to Real-Imag/1

== system Diode_Clamped_Multilevel_Inverter/Induction Machine Model/Park transform1 ==
  In1 : Inport
  phi : Inport  Port=2
  Complex to Real-Imag : ComplexToRealImag
  Constant : Constant  Value=-pi/2
  Cos+jSin : Trigonometry  Operator=cos + jsin
  Display : Display
  Gain : Gain  Gain=-1
  Product : Product
  Sum : Sum  Inputs=|++
  Vrd : Outport
  Vrq : Outport  Port=2
  wires:
  In1/1 -> Product/1  "alpha-beta"
  Cos+jSin/1 -> Product/2, Display/1
  Gain/1 -> Cos+jSin/1
  Product/1 -> Complex to Real-Imag/1
  Complex to Real-Imag/1 -> Vrd/1  "d-axis"
  Complex to Real-Imag/2 -> Vrq/1  "q-axis"
  phi/1 -> Sum/1
  Sum/1 -> Gain/1
  Constant/1 -> Sum/2

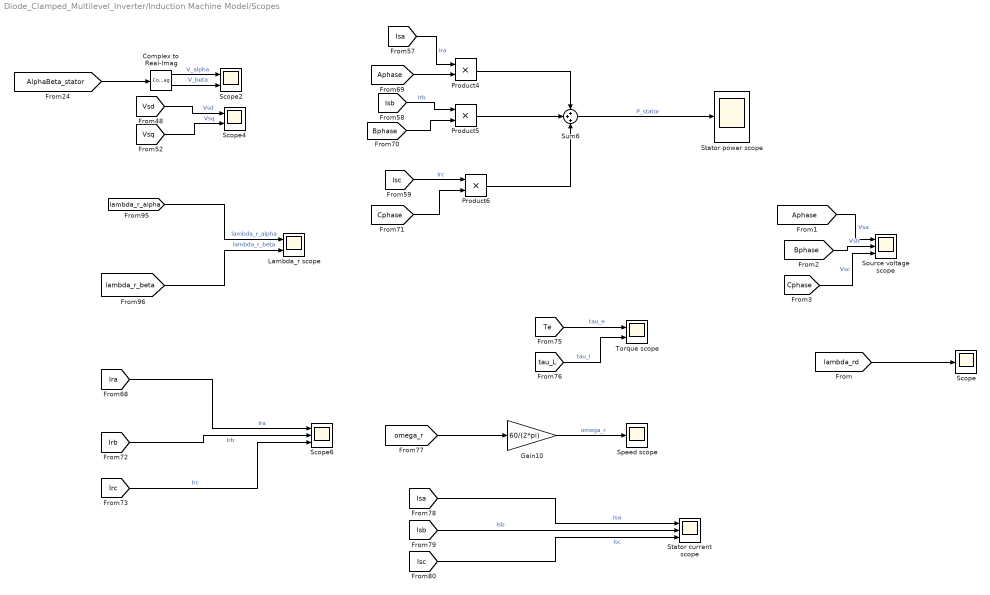
== system Diode_Clamped_Multilevel_Inverter/Induction Machine Model/Scopes ==
  Complex to Real-Imag : ComplexToRealImag
  Gain10 : Gain  Gain=60/(2*pi)
  Lambda_r scope : Scope  NumInputPorts=2
  Product4 : Product
  Product5 : Product
  Product6 : Product
  Scope : Scope
  Scope2 : Scope  NumInputPorts=2
  Scope4 : Scope  NumInputPorts=2
  Scope6 : Scope  NumInputPorts=3
  Source voltage scope : Scope  NumInputPorts=3
  Speed scope : Scope
  Stator current scope : Scope  NumInputPorts=3
  Stator power scope : Scope
  Sum6 : Sum  Inputs=+++
  Torque scope : Scope  NumInputPorts=2
  wires:
  [tau_L] -> Torque scope/2  "tau_l"
  Product4/1 -> Sum6/1
  Product5/1 -> Sum6/2
  [Isb] -> Stator current scope/2  "Isb"
  [Bphase] -> Product5/2
  [Irc] -> Scope6/3  "Irc"
  [Irb] -> Scope6/2  "Irb"
  [lambda_r_alpha] -> Lambda_r scope/1  "lambda_r_alpha"
  [Isb] -> Product5/1  "Irb"
  [Te] -> Torque scope/1  "tau_e"
  [lambda_r_beta] -> Lambda_r scope/2  "lambda_r_beta"
  [omega_r] -> Gain10/1
  Gain10/1 -> Speed scope/1  "omega_r"
  [Isc] -> Stator current scope/3  "Isc"
  [Isc] -> Product6/1  "Irc"
  Sum6/1 -> Stator power scope/1  "P_stator"
  [Isa] -> Stator current scope/1  "Isa"
  [Ira] -> Scope6/1  "Ira"
  [Aphase] -> Product4/2
  [Cphase] -> Product6/2
  [Isa] -> Product4/1  "Ira"
  Product6/1 -> Sum6/3
  [Aphase] -> Source voltage scope/1  "Vsa"
  [Cphase] -> Source voltage scope/3  "Vsc"
  [Bphase] -> Source voltage scope/2  "Vsb"
  [AlphaBeta_stator] -> Complex to Real-Imag/1
  Complex to Real-Imag/2 -> Scope2/2  "V_beta"
  Complex to Real-Imag/1 -> Scope2/1  "V_alpha"
  [Vsd] -> Scope4/1  "Vsd"
  [Vsq] -> Scope4/2  "Vsq"
  [lambda_rd] -> Scope/1

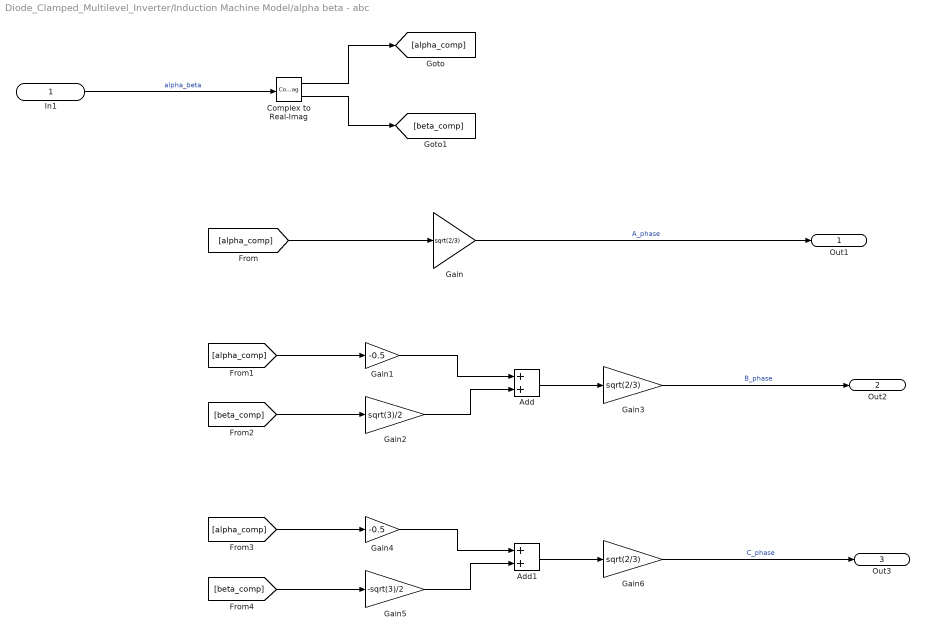
== system Diode_Clamped_Multilevel_Inverter/Induction Machine Model/alpha beta - abc ==
  In1 : Inport
  Add : Sum
  Add1 : Sum
  Complex to Real-Imag : ComplexToRealImag
  Gain : Gain  Gain=sqrt(2/3)
  Gain1 : Gain  Gain=-0.5
  Gain2 : Gain  Gain=sqrt(3)/2
  Gain3 : Gain  Gain=sqrt(2/3)
  Gain4 : Gain  Gain=-0.5
  Gain5 : Gain  Gain=-sqrt(3)/2
  Gain6 : Gain  Gain=sqrt(2/3)
  Out1 : Outport
  Out2 : Outport  Port=2
  Out3 : Outport  Port=3
  wires:
  In1/1 -> Complex to Real-Imag/1  "alpha_beta"
  Complex to Real-Imag/1 -> [alpha_comp]
  Complex to Real-Imag/2 -> [beta_comp]
  Gain/1 -> Out1/1  "A_phase"
  [alpha_comp] -> Gain/1
  [alpha_comp] -> Gain1/1
  [beta_comp] -> Gain2/1
  Gain1/1 -> Add/1
  Gain2/1 -> Add/2
  Add/1 -> Gain3/1
  Gain3/1 -> Out2/1  "B_phase"
  Add1/1 -> Gain6/1
  Gain6/1 -> Out3/1  "C_phase"
  Gain4/1 -> Add1/1
  [beta_comp] -> Gain5/1
  Gain5/1 -> Add1/2
  [alpha_comp] -> Gain4/1

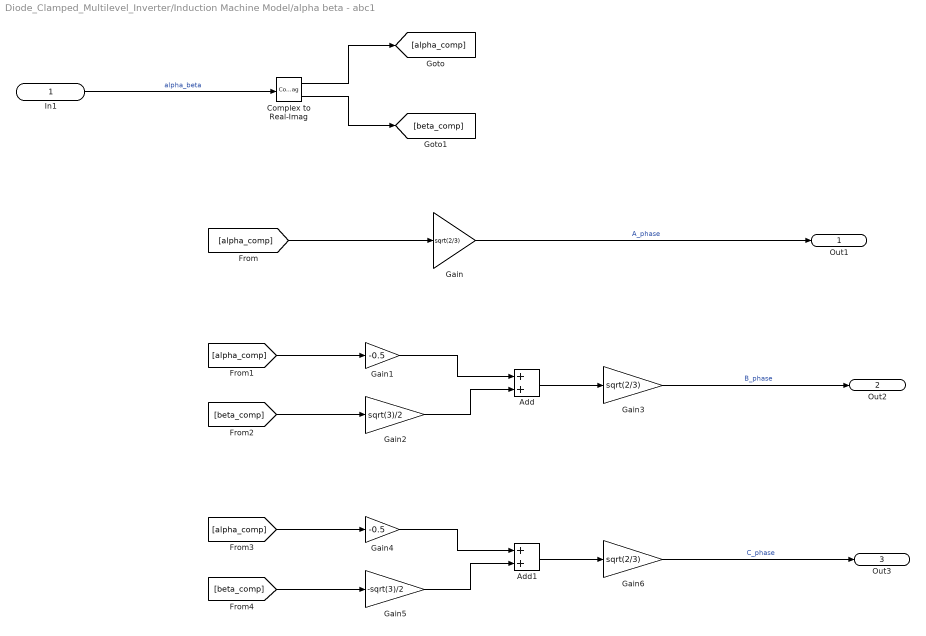
== system Diode_Clamped_Multilevel_Inverter/Induction Machine Model/alpha beta - abc1 ==
  In1 : Inport
  Add : Sum
  Add1 : Sum
  Complex to Real-Imag : ComplexToRealImag
  Gain : Gain  Gain=sqrt(2/3)
  Gain1 : Gain  Gain=-0.5
  Gain2 : Gain  Gain=sqrt(3)/2
  Gain3 : Gain  Gain=sqrt(2/3)
  Gain4 : Gain  Gain=-0.5
  Gain5 : Gain  Gain=-sqrt(3)/2
  Gain6 : Gain  Gain=sqrt(2/3)
  Out1 : Outport
  Out2 : Outport  Port=2
  Out3 : Outport  Port=3
  wires:
  In1/1 -> Complex to Real-Imag/1  "alpha_beta"
  Complex to Real-Imag/1 -> [alpha_comp]
  Complex to Real-Imag/2 -> [beta_comp]
  Gain/1 -> Out1/1  "A_phase"
  [alpha_comp] -> Gain/1
  [alpha_comp] -> Gain1/1
  [beta_comp] -> Gain2/1
  Gain1/1 -> Add/1
  Gain2/1 -> Add/2
  Add/1 -> Gain3/1
  Gain3/1 -> Out2/1  "B_phase"
  Add1/1 -> Gain6/1
  Gain6/1 -> Out3/1  "C_phase"
  Gain4/1 -> Add1/1
  [beta_comp] -> Gain5/1
  Gain5/1 -> Add1/2
  [alpha_comp] -> Gain4/1

== system Diode_Clamped_Multilevel_Inverter/Induction Machine Model/dq-alpha beta ==
  d-axis : Inport
  q-axis : Inport  Port=2
  In3 : Inport  Port=3
  Constant : Constant  Value=-pi/2
  Cos+jSin : Trigonometry  Operator=cos + jsin
  Product : Product
  Real-Imag to Complex : RealImagToComplex
  Sum : Sum  Inputs=|++
  Out1 : Outport
  wires:
  d-axis/1 -> Real-Imag to Complex/1  "d-axis"
  q-axis/1 -> Real-Imag to Complex/2  "q-axis"
  Real-Imag to Complex/1 -> Product/1
  Cos+jSin/1 -> Product/2
  Product/1 -> Out1/1  "alpha_beta"
  In3/1 -> Sum/1  "theta"
  Sum/1 -> Cos+jSin/1
  Constant/1 -> Sum/2

== system Diode_Clamped_Multilevel_Inverter/Induction Machine Model/dq-alpha beta1 ==
  d-axis : Inport
  q-axis : Inport  Port=2
  In1 : Inport  Port=3
  Constant : Constant  Value=-pi/2
  Cos+jSin : Trigonometry  Operator=cos + jsin
  Product : Product
  Real-Imag to Complex : RealImagToComplex
  Sum : Sum  Inputs=|++
  Out1 : Outport
  wires:
  d-axis/1 -> Real-Imag to Complex/1  "d-axis"
  q-axis/1 -> Real-Imag to Complex/2  "q-axis"
  Real-Imag to Complex/1 -> Product/1
  Cos+jSin/1 -> Product/2
  Product/1 -> Out1/1  "alpha_beta"
  In1/1 -> Sum/1  "theta"
  Constant/1 -> Sum/2
  Sum/1 -> Cos+jSin/1

== system Diode_Clamped_Multilevel_Inverter/Induction Machine Model/dq-alpha beta2 ==
  d-axis : Inport
  q-axis : Inport  Port=2
  In3 : Inport  Port=3
  Constant : Constant  Value=-pi/2
  Cos+jSin : Trigonometry  Operator=cos + jsin
  Product : Product
  Real-Imag to Complex : RealImagToComplex
  Sum : Sum  Inputs=|++
  Out1 : Outport
  wires:
  d-axis/1 -> Real-Imag to Complex/1  "d-axis"
  q-axis/1 -> Real-Imag to Complex/2  "q-axis"
  Real-Imag to Complex/1 -> Product/1
  Cos+jSin/1 -> Product/2
  Product/1 -> Out1/1  "alpha_beta"
  In3/1 -> Sum/1  "theta"
  Sum/1 -> Cos+jSin/1
  Constant/1 -> Sum/2

== system Diode_Clamped_Multilevel_Inverter/Induction Machine Model/dq-alpha beta3 ==
  d-axis : Inport
  q-axis : Inport  Port=2
  In3 : Inport  Port=3
  Constant : Constant  Value=-pi/2
  Cos+jSin : Trigonometry  Operator=cos + jsin
  Product : Product
  Real-Imag to Complex : RealImagToComplex
  Sum : Sum  Inputs=|++
  Out1 : Outport
  wires:
  d-axis/1 -> Real-Imag to Complex/1  "d-axis"
  q-axis/1 -> Real-Imag to Complex/2  "q-axis"
  Real-Imag to Complex/1 -> Product/1
  Cos+jSin/1 -> Product/2
  Product/1 -> Out1/1  "alpha_beta"
  In3/1 -> Sum/1  "theta"
  Sum/1 -> Cos+jSin/1
  Constant/1 -> Sum/2

== system Diode_Clamped_Multilevel_Inverter/Induction Machine Model/dq-alpha beta4 ==
  d-axis : Inport
  q-axis : Inport  Port=2
  In3 : Inport  Port=3
  Constant : Constant  Value=-pi/2
  Cos+jSin : Trigonometry  Operator=cos + jsin
  Product : Product
  Real-Imag to Complex : RealImagToComplex
  Sum : Sum  Inputs=|++
  Out1 : Outport
  wires:
  d-axis/1 -> Real-Imag to Complex/1  "d-axis"
  q-axis/1 -> Real-Imag to Complex/2  "q-axis"
  Real-Imag to Complex/1 -> Product/1
  Cos+jSin/1 -> Product/2
  Product/1 -> Out1/1  "alpha_beta"
  In3/1 -> Sum/1  "theta"
  Sum/1 -> Cos+jSin/1
  Constant/1 -> Sum/2

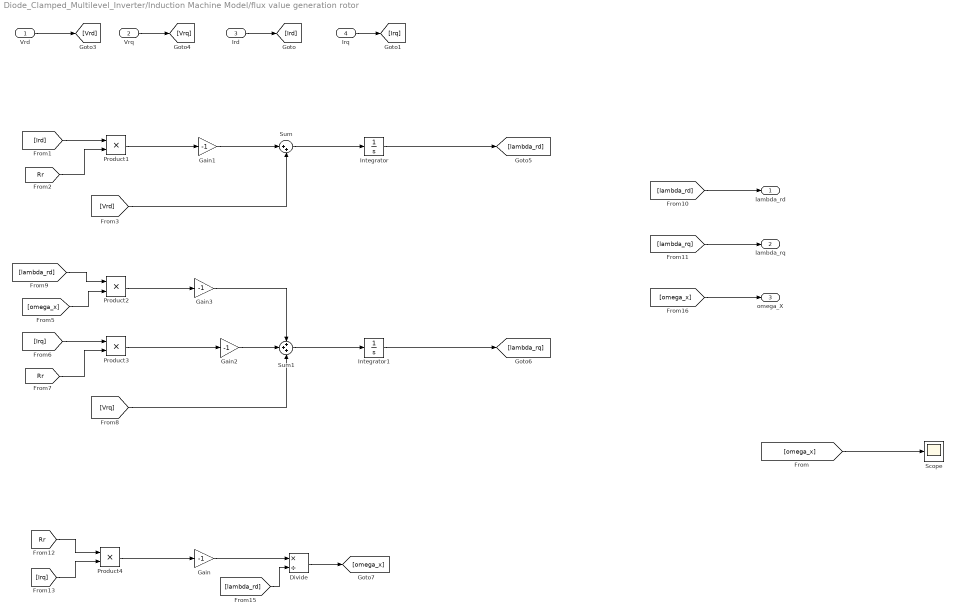
== system Diode_Clamped_Multilevel_Inverter/Induction Machine Model/flux value generation rotor ==
  Vrd : Inport
  Vrq : Inport  Port=2
  Ird : Inport  Port=3
  Irq : Inport  Port=4
  Divide : Product  Inputs=*/
  Gain{,1..3} (4 alike) : Gain  Gain=-1
  Integrator : Integrator  InitialCondition=1e-5
  Integrator1 : Integrator  InitialCondition=1e-5
  Product{1..4} (4 alike) : Product
  Scope : Scope
  Sum : Sum  Inputs=|++
  Sum1 : Sum  Inputs=+++
  lambda_rd : Outport
  lambda_rq : Outport  Port=2
  omega_X : Outport  Port=3
  wires:
  Ird/1 -> [Ird]
  Irq/1 -> [Irq]
  Vrd/1 -> [Vrd]
  Vrq/1 -> [Vrq]
  [Ird] -> Product1/1
  [Rr] -> Product1/2
  Product1/1 -> Gain1/1
  Sum/1 -> Integrator/1
  Integrator/1 -> [lambda_rd]
  [lambda_rd] -> Product2/1
  Sum1/1 -> Integrator1/1
  Product3/1 -> Gain2/1
  [Irq] -> Product3/1
  [Vrq] -> Sum1/3
  [omega_x] -> Product2/2
  [Rr] -> Product3/2
  Product2/1 -> Gain3/1
  Gain2/1 -> Sum1/2
  [lambda_rd] -> lambda_rd/1
  [lambda_rq] -> lambda_rq/1
  [Rr] -> Product4/1
  [Irq] -> Product4/2
  [lambda_rd] -> Divide/2
  Divide/1 -> [omega_x]
  [omega_x] -> omega_X/1
  Integrator1/1 -> [lambda_rq]
  Gain1/1 -> Sum/1
  [Vrd] -> Sum/2
  Product4/1 -> Gain/1
  Gain/1 -> Divide/1
  Gain3/1 -> Sum1/1
  [omega_x] -> Scope/1

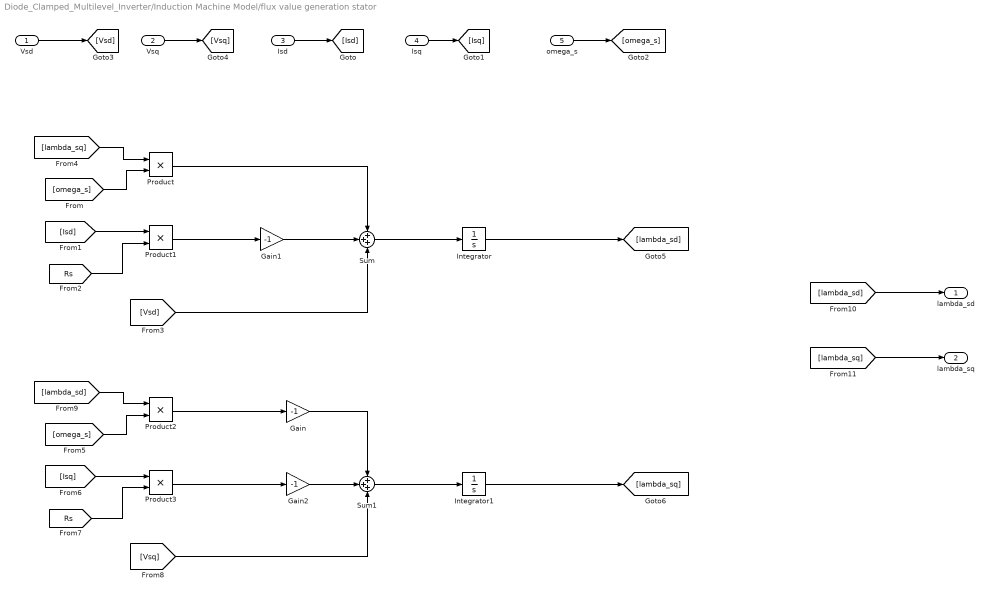
== system Diode_Clamped_Multilevel_Inverter/Induction Machine Model/flux value generation stator ==
  Vsd : Inport
  Vsq : Inport  Port=2
  Isd : Inport  Port=3
  Isq : Inport  Port=4
  omega_s : Inport  Port=5
  Gain : Gain  Gain=-1
  Gain1 : Gain  Gain=-1
  Gain2 : Gain  Gain=-1
  Integrator : Integrator
  Integrator1 : Integrator
  Product{,1..3} (4 alike) : Product
  Sum : Sum  Inputs=+++
  Sum1 : Sum  Inputs=+++
  lambda_sd : Outport
  lambda_sq : Outport  Port=2
  wires:
  Isd/1 -> [Isd]
  Isq/1 -> [Isq]
  omega_s/1 -> [omega_s]
  Vsd/1 -> [Vsd]
  Vsq/1 -> [Vsq]
  [omega_s] -> Product/2
  [Isd] -> Product1/1
  [Rs] -> Product1/2
  Product1/1 -> Gain1/1
  Product/1 -> Sum/1
  [Vsd] -> Sum/3
  Sum/1 -> Integrator/1
  Integrator/1 -> [lambda_sd]
  [lambda_sq] -> Product/1
  [lambda_sd] -> Product2/1
  Sum1/1 -> Integrator1/1
  Integrator1/1 -> [lambda_sq]
  Product3/1 -> Gain2/1
  Product2/1 -> Gain/1
  [Isq] -> Product3/1
  [Vsq] -> Sum1/3
  [omega_s] -> Product2/2
  [Rs] -> Product3/2
  Gain/1 -> Sum1/1
  Gain1/1 -> Sum/2
  Gain2/1 -> Sum1/2
  [lambda_sd] -> lambda_sd/1
  [lambda_sq] -> lambda_sq/1
